simulink model "ex3TF_SS"  (R2014b)
settings: Solver=ode45  StartTime=0.0  StopTime=10.0  RelTol=1e-3
settings Model: Creator=99641  LastModifiedBy=99641

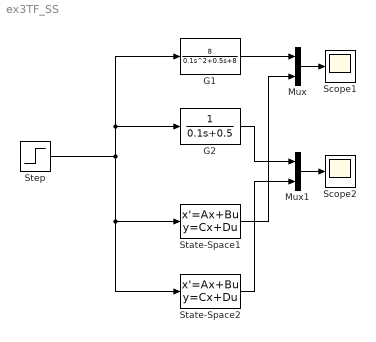
== system ex3TF_SS ==
  G1 : TransferFcn  Numerator=8  Denominator=[0.1,0.5,8]
  "G2 " : TransferFcn  Numerator=1  Denominator=[0.1,0.5]
  Mux : Mux  Inputs=2
  Mux1 : Mux  Inputs=2
  Scope1 : Scope
  Scope2 : Scope
  State-Space1 : StateSpace  A=[-5,-10;8,0]  B=[4;0]  C=[0,2.5]  D=0  X0=0
  State-Space2 : StateSpace  A=-5  B=4  C=2.5  D=0  X0=0
  Step : Step  SampleTime=0
  wires:
  State-Space1/1 -> Mux/2
  Mux/1 -> Scope1/1
  G1/1 -> Mux/1
  Mux1/1 -> Scope2/1
  "G2 "/1 -> Mux1/1
  State-Space2/1 -> Mux1/2
  Step/1 -> State-Space2/1, State-Space1/1, "G2 "/1, G1/1
